simulink model "MIL_Simulation"  (R2022b)
settings: configuration reference "MIL_Simulation_ConfigSet_UDEMY" (kept outside this file)
PreLoadFcn:
  | run_start;
undefined symbols (not defined in the file or in its folder): DiscIntNeverNeededParam, KI_w, Kp_w, rad_s_to_rpm, sigbuilder_block, T_limit_Nm, w_cntrl_reset, w_m_max
libraries: simulink x2
settings Model: DataDictionary=FieldOrientedControl_UDEMY.sldd  Creator=Markez  LastModifiedBy=Musaab
settings ConfigSetRef: SourceName=MIL_Simulation_ConfigSet_UDEMY

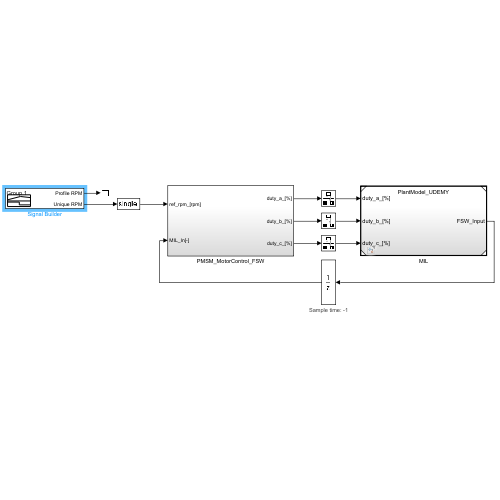
[thumbnail: Simulink's stored preview of the top-level diagram]
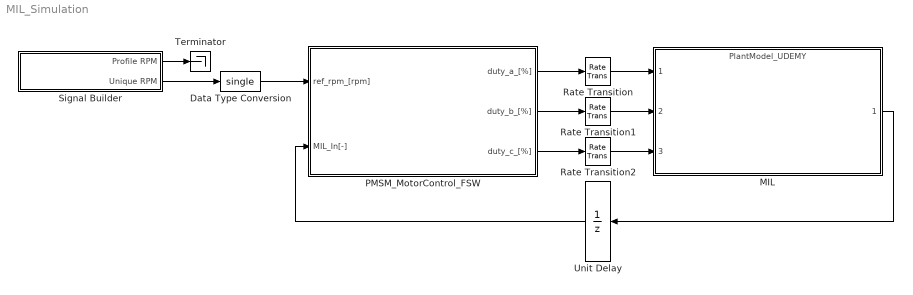
== system MIL_Simulation ==
  Data Type Conversion : DataTypeConversion  OutDataTypeStr=single  RndMeth=Simplest
  MIL : ModelReference  ModelNameDialog=PlantModel_UDEMY.slx  SimulationMode=Normal  ModelReferenceVersion=1.9
  PMSM_MotorControl_FSW : Subsystem
  Rate Transition : RateTransition  OutPortSampleTime=sample_time_MIL
  Rate Transition1 : RateTransition  OutPortSampleTime=sample_time_MIL
  Rate Transition2 : RateTransition  OutPortSampleTime=sample_time_MIL
  Signal Builder : Subsystem  Tag=STV Subsys  LoadFcn=sigbuilder_block('load',[715.5 30.75 718.5 648 ]);  StartFcn=sigbuilder_block('start');  StopFcn=sigbuilder_block('stop');  ClipboardFcn=sigbuilder_block('clipboard');  mask(Sigbuilder block){tuvar=[0:10]}
      mask help: Simulink:masks:SigbuilderBlock_MD
      mask init:
      | if ~strcmp(get_param(bdroot(gcbh),'SimulationStatus'),'stopped') tuvar = sigbuilder_block('maskInit'); end
      settings: CopyFcn=sigbuilder_block('copy');  DeleteFcn=sigbuilder_block('delete');  ModelCloseFcn=sigbuilder_block('modelClose');  PreSaveFcn=sigbuilder_block('preSave');  PauseFcn=sigbuilder_block('pause');  ContinueFcn=sigbuilder_block('continue');  NameChangeFcn=sigbuilder_block('namechange');  OpenFcn=sigbuilder_block('open',[715.5 30.75 718.5 648 ]);  CloseFcn=sigbuilder_block('close');
      mask Display: plot(0, 0, 100, 100,[2, 2, 32, 32, 2], [68, 8, 8, 68, 68],[32, 2], [38, 38], [32, 19, 2],[53, 60, 44], [32, 17, 17, 2],[16, 16, 31, 31]);txt = getActiveGroup(gcbh);text(2, 100, txt,'verticalAlignment', 'top');
  Terminator : Terminator
  Unit Delay : UnitDelay  SampleTime=-1  HasFrameUpgradeWarning=on
      settings: AttributesFormatString=Sample time: %<SampleTime>
  wires:
  MIL/1 -> Unit Delay/1
  PMSM_MotorControl_FSW/2(duty_b_[%]) -> Rate Transition1/1
  Rate Transition2/1 -> MIL/3
  PMSM_MotorControl_FSW/1(duty_a_[%]) -> Rate Transition/1
  Unit Delay/1 -> PMSM_MotorControl_FSW/2(MIL_In[-])
  PMSM_MotorControl_FSW/3(duty_c_[%]) -> Rate Transition2/1
  Signal Builder/2(Unique RPM) -> Data Type Conversion/1
  Signal Builder/1(Profile RPM) -> Terminator/1
  Data Type Conversion/1 -> PMSM_MotorControl_FSW/1(ref_rpm_[rpm])
  Rate Transition/1 -> MIL/1
  Rate Transition1/1 -> MIL/2

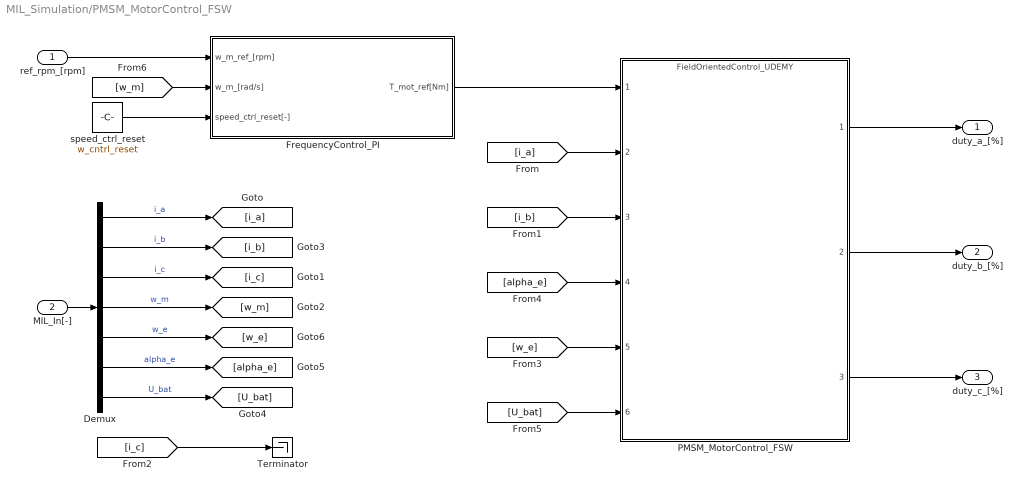
== system MIL_Simulation/PMSM_MotorControl_FSW ==
  ref_rpm_[rpm] : Inport
  MIL_In[-] : Inport  Port=2
  Demux : Demux  Outputs=7
  FrequencyControl_PI : Subsystem
  PMSM_MotorControl_FSW : ModelReference  ModelNameDialog=FieldOrientedControl_UDEMY.slx  SimulationMode=Normal  ModelReferenceVersion=3.8
  Terminator : Terminator
  speed_ctrl_reset : Constant  Value=w_cntrl_reset  OutDataTypeStr=boolean
  duty_a_[%] : Outport  OutDataTypeStr=single
  duty_b_[%] : Outport  Port=2  OutDataTypeStr=single
  duty_c_[%] : Outport  Port=3  OutDataTypeStr=single
  wires:
  PMSM_MotorControl_FSW/1 -> duty_a_[%]/1
  PMSM_MotorControl_FSW/2 -> duty_b_[%]/1
  PMSM_MotorControl_FSW/3 -> duty_c_[%]/1
  FrequencyControl_PI/1(T_mot_ref[Nm]) -> PMSM_MotorControl_FSW/1
  ref_rpm_[rpm]/1 -> FrequencyControl_PI/1(w_m_ref_[rpm])
  speed_ctrl_reset/1 -> FrequencyControl_PI/3(speed_ctrl_reset[-])
  MIL_In[-]/1 -> Demux/1
  Demux/1 -> [i_a]  "i_a"
  Demux/3 -> [i_c]  "i_c"
  Demux/2 -> [i_b]  "i_b"
  Demux/4 -> [w_m]  "w_m"
  [i_a] -> PMSM_MotorControl_FSW/2
  [i_b] -> PMSM_MotorControl_FSW/3
  [i_c] -> Terminator/1
  [w_e] -> PMSM_MotorControl_FSW/5
  [alpha_e] -> PMSM_MotorControl_FSW/4
  [U_bat] -> PMSM_MotorControl_FSW/6
  [w_m] -> FrequencyControl_PI/2(w_m_[rad/s])
  Demux/7 -> [U_bat]  "U_bat"
  Demux/6 -> [alpha_e]  "alpha_e"
  Demux/5 -> [w_e]  "w_e"

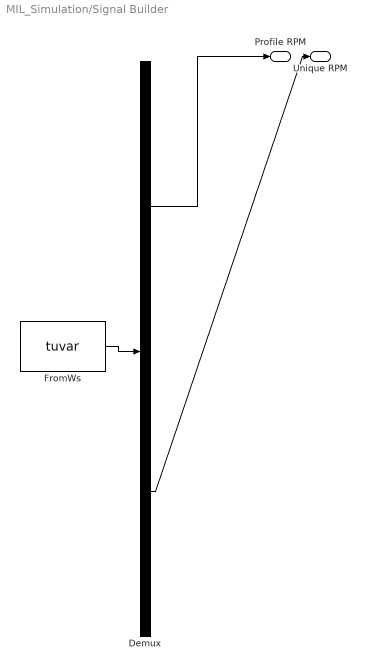
== system MIL_Simulation/Signal Builder ==
  Demux : Demux  Tag=STV Demux  Outputs=2
      settings: DisplayOption=none
  FromWs : FromWorkspace  Tag=STV FromWs  VariableName=tuvar
      SigBuilderData=|
      | common.afterFinalStr = 'Extrapolate'
      | common.sampleTime = 0
      | dataSet.timeRange = [0 1.5]
      | dataSet.name = 'Group 1'
      | sbobj.Groups.Name = 'Group 1'
      | sbobj.Groups.Signals(1).Name = 'Profile RPM'
      | sbobj.Groups.Signals(1).XData = [0 0.015 0.5 0.8 1.3 1.5]
      | sbobj.Groups.Signals(1).YData = [0 0 6000 6000 0 0]
      | sbobj.Groups.Signals(2).Name = 'Unique RPM'
      | sbobj.Groups.Signals(2).XData = [0 0.015 0.015 1 1 1.5]
      | sbobj.Groups.Signals(2).YData = [0 0 6000 6000 0 0]
      | sbobj.Groups.TimeRange = [0 1.5]
  Profile RPM : Outport  Tag=STV Outport
  Unique RPM : Outport  Tag=STV Outport  Port=2
  wires:
  FromWs/1 -> Demux/1
  Demux/1 -> Profile RPM/1
  Demux/2 -> Unique RPM/1

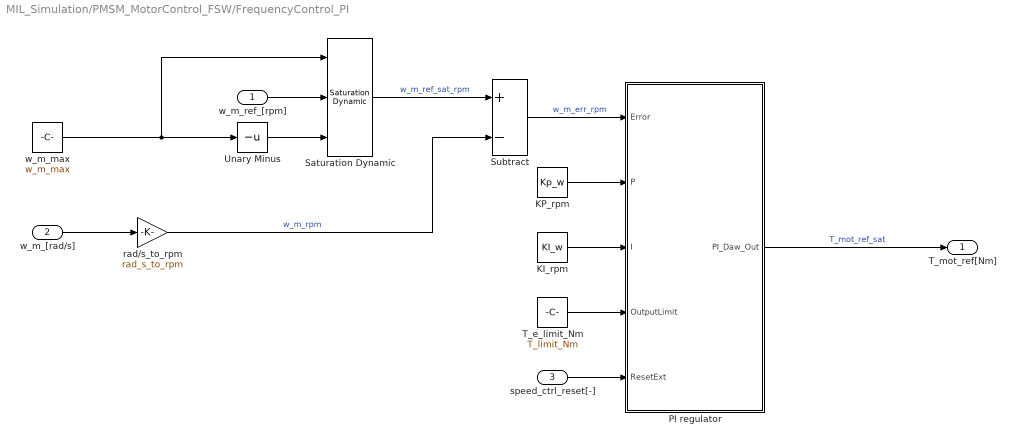
== system MIL_Simulation/PMSM_MotorControl_FSW/FrequencyControl_PI ==
  w_m_ref_[rpm] : Inport
  w_m_[rad/s] : Inport  Port=2
  speed_ctrl_reset[-] : Inport  Port=3
  KI_rpm : Constant  Value=KI_w  OutDataTypeStr=single
  KP_rpm : Constant  Value=Kp_w  OutDataTypeStr=single
  PI regulator : Subsystem
  Saturation Dynamic : simulink/Discontinuities/Saturation Dynamic  OutMin=[]  OutMax=[]  OutDataTypeStr=Inherit: Same as second input  OutDataType=fixdt(1, 16)  OutScaling=2^-10  RndMeth=Simplest  DoSatur=off
  Subtract : Sum  Inputs=+-  RndMeth=Simplest  SaturateOnIntegerOverflow=on
  T_e_limit_Nm : Constant  Value=T_limit_Nm
  Unary Minus : UnaryMinus  SaturateOnIntegerOverflow=on
  rad/s_to_rpm : Gain  Gain=rad_s_to_rpm  RndMeth=Simplest  SaturateOnIntegerOverflow=on
  w_m_max : Constant  Value=w_m_max
  T_mot_ref[Nm] : Outport
  wires:
  KI_rpm/1 -> PI regulator/3(I)
  KP_rpm/1 -> PI regulator/2(P)
  w_m_max/1 -> Saturation Dynamic/1, Unary Minus/1
  T_e_limit_Nm/1 -> PI regulator/4(OutputLimit)
  w_m_ref_[rpm]/1 -> Saturation Dynamic/2
  PI regulator/1(PI_Daw_Out) -> T_mot_ref[Nm]/1  "T_mot_ref_sat"
  speed_ctrl_reset[-]/1 -> PI regulator/5(ResetExt)
  Saturation Dynamic/1 -> Subtract/1  "w_m_ref_sat_rpm"
  Subtract/1 -> PI regulator/1(Error)  "w_m_err_rpm"
  Unary Minus/1 -> Saturation Dynamic/3
  w_m_[rad/s]/1 -> rad/s_to_rpm/1
  rad/s_to_rpm/1 -> Subtract/2  "w_m_rpm"

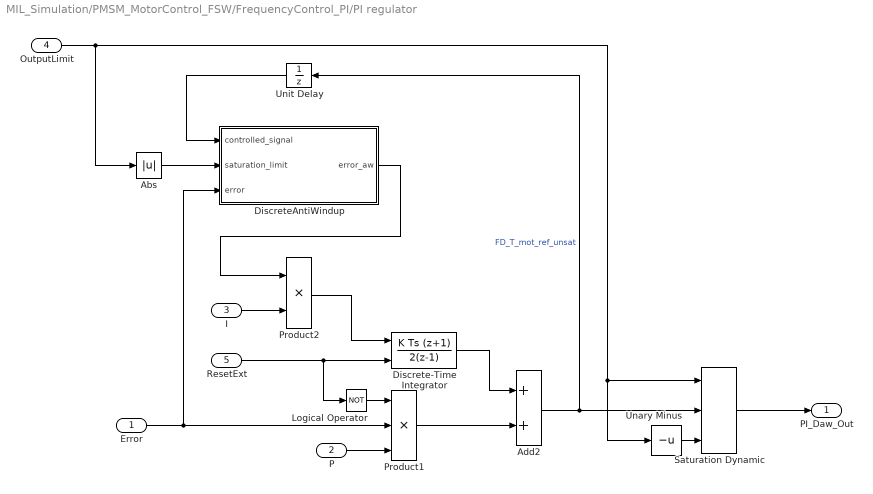
== system MIL_Simulation/PMSM_MotorControl_FSW/FrequencyControl_PI/PI regulator ==
  Error : Inport
  P : Inport  Port=2
  I : Inport  Port=3
  OutputLimit : Inport  Port=4
  ResetExt : Inport  Port=5
  Abs : Abs  RndMeth=Simplest
  Add2 : Sum  RndMeth=Simplest  SaturateOnIntegerOverflow=on
  Discrete-Time Integrator : DiscreteIntegrator  IntegratorMethod=Integration: Trapezoidal  ExternalReset=level  SampleTime=-1  RndMeth=Simplest  SaturateOnIntegerOverflow=on  ICPrevOutput=DiscIntNeverNeededParam  ICPrevScaledInput=DiscIntNeverNeededParam
  DiscreteAntiWindup : Subsystem
  Logical Operator : Logic  Operator=NOT  AllPortsSameDT=off  OutDataTypeStr=boolean
  Product1 : Product  Inputs=3  RndMeth=Simplest  SaturateOnIntegerOverflow=on
  Product2 : Product  RndMeth=Simplest  SaturateOnIntegerOverflow=on
  Saturation Dynamic : simulink/Discontinuities/Saturation Dynamic  OutMin=[]  OutMax=[]  OutDataTypeStr=Inherit: Same as second input  OutDataType=fixdt(1, 16)  OutScaling=2^-10  RndMeth=Simplest  DoSatur=off
  Unary Minus : UnaryMinus  SaturateOnIntegerOverflow=on
  Unit Delay : UnitDelay  SampleTime=-1  HasFrameUpgradeWarning=on
      settings: AttributesFormatString=Sample time: %<SampleTime>
  PI_Daw_Out : Outport
  wires:
  Unary Minus/1 -> Saturation Dynamic/3
  Unit Delay/1 -> DiscreteAntiWindup/1(controlled_signal)
  P/1 -> Product1/3
  Discrete-Time Integrator/1 -> Add2/1
  ResetExt/1 -> Logical Operator/1, Discrete-Time Integrator/2
  Saturation Dynamic/1 -> PI_Daw_Out/1
  Product1/1 -> Add2/2
  Error/1 -> Product1/2, DiscreteAntiWindup/3(error)
  OutputLimit/1 -> Unary Minus/1, Saturation Dynamic/1, Abs/1
  Add2/1 -> Saturation Dynamic/2, Unit Delay/1  "FD_T_mot_ref_unsat"
  Abs/1 -> DiscreteAntiWindup/2("saturation_limit ")
  DiscreteAntiWindup/1(error_aw) -> Product2/1
  Product2/1 -> Discrete-Time Integrator/1
  I/1 -> Product2/2
  Logical Operator/1 -> Product1/1

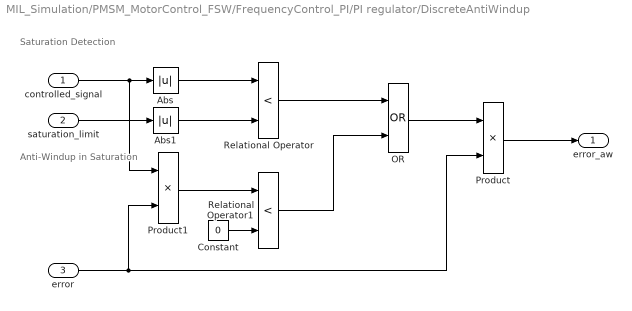
== system MIL_Simulation/PMSM_MotorControl_FSW/FrequencyControl_PI/PI regulator/DiscreteAntiWindup ==
  note: Saturation Detection
  note: Anti-Windup in Saturation
  controlled_signal : Inport
  "saturation_limit " : Inport  Port=2
  error : Inport  Port=3
  Abs : Abs  RndMeth=Simplest
  Abs1 : Abs  RndMeth=Simplest
  Constant : Constant  Value=0  OutDataTypeStr=single
  OR : Logic  Operator=OR  AllPortsSameDT=off  OutDataTypeStr=boolean
  Product : Product  RndMeth=Simplest  SaturateOnIntegerOverflow=on
  Product1 : Product  RndMeth=Simplest  SaturateOnIntegerOverflow=on
  Relational Operator : RelationalOperator  Operator=<  OutDataTypeStr=boolean  RndMeth=Simplest  InputSameDT=off
  Relational Operator1 : RelationalOperator  Operator=<  OutDataTypeStr=boolean  RndMeth=Simplest  InputSameDT=off
  error_aw : Outport
  wires:
  Relational Operator1/1 -> OR/2
  Constant/1 -> Relational Operator1/2
  Product1/1 -> Relational Operator1/1
  Product/1 -> error_aw/1
  error/1 -> Product/2, Product1/2
  OR/1 -> Product/1
  Relational Operator/1 -> OR/1
  Abs/1 -> Relational Operator/1
  Abs1/1 -> Relational Operator/2
  "saturation_limit "/1 -> Abs1/1
  controlled_signal/1 -> Abs/1, Product1/1
